simulink model "activity2_df1_uncorrected"  (R2024b)
settings: Solver=FixedStepAuto  StartTime=0.0  StopTime=10.0  FixedStep=1/44100  RelTol=1e-3
libraries: dspsnks4 x1, dspvision x1
settings Model: Creator=ck  LastModifiedBy=ck

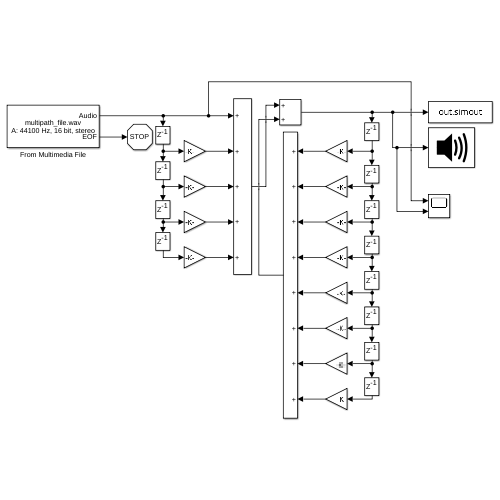
[thumbnail: Simulink's stored preview of the top-level diagram]
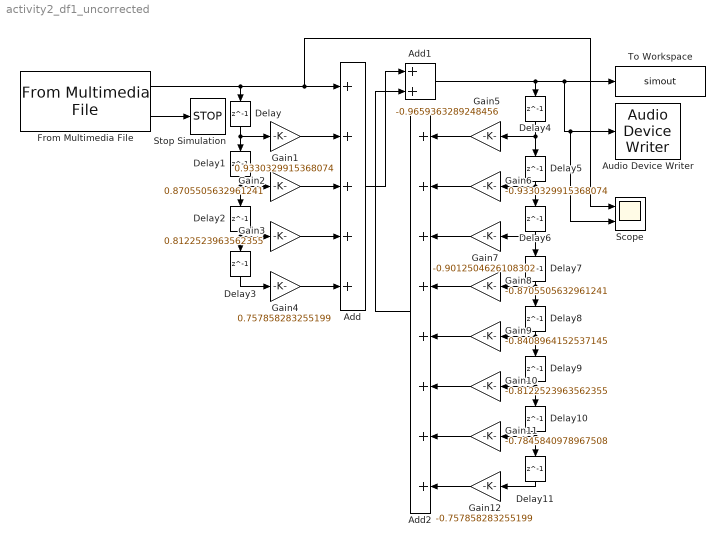
== system activity2_df1_uncorrected ==
  Add : Sum  Inputs=+++++
  Add1 : Sum
  Add2 : Sum  Inputs=++++++++
  Audio Device Writer : dspsnks4/Audio Device Writer  Driver=ALSA  Device=Default  InheritSampleRate=on  SampleRate=44100  BitDepth=16-bit integer  BufferSize=4096  NumBuffers=10  DefaultOutputChannelMapping=on  OutputChannelMapping=1:2  OutputNumUnderrunSamples=off  DriverIdx=8  DeviceWarnFlag=''
  Delay{,1..11} (12 alike) : Delay  DelayLength=1  InitialCondition=0
  From Multimedia File : dspvision/From Multimedia File  inputFilename=/home/ck/Documents/ece164/multipath_file.wav  readRange=[1 Inf]  loop=on  numPlays=inf  outputStreams=Audio only  videoDataType=single  audioDataType=double  inheritSampleTime=on  userDefinedSampleTime=1/30  noAudioOutput=off  isIntensityVideo=off  fourcc=RGB  colorVideoFormat=One multidimensional signal  outputEOF=on  dataOrg=Column-major  audioFrameSize=1  computeAudioFrameSize=off  outSamplingMode=Sample based
      settings: LibrarySourceBlock=dspsrcs4/From Multimedia File
  Gain1 : Gain  Gain=0.9330329915368074
  Gain10 : Gain  Gain=-0.8122523963562355
  Gain11 : Gain  Gain=-0.7845840978967508
  Gain12 : Gain  Gain=-0.757858283255199
  Gain2 : Gain  Gain=0.8705505632961241
  Gain3 : Gain  Gain=0.8122523963562355
  Gain4 : Gain  Gain=0.757858283255199
  Gain5 : Gain  Gain=-0.9659363289248456
  Gain6 : Gain  Gain=-0.9330329915368074
  Gain7 : Gain  Gain=-0.9012504626108302
  Gain8 : Gain  Gain=-0.8705505632961241
  Gain9 : Gain  Gain=-0.8408964152537145
  Scope : Scope  NumInputPorts=2
  Stop Simulation : Stop
  To Workspace : ToWorkspace  VariableName=simout  SaveFormat=Timeseries  SampleTime=-1
  wires:
  From Multimedia File/2 -> Stop Simulation/1
  From Multimedia File/1 -> Scope/1, Add/1, Delay/1
  Add/1 -> Add1/1
  Gain1/1 -> Add/2
  Gain2/1 -> Add/3
  Gain3/1 -> Add/4
  Gain4/1 -> Add/5
  Delay/1 -> Gain1/1, Delay1/1
  Delay1/1 -> Gain2/1, Delay2/1
  Delay2/1 -> Gain3/1, Delay3/1
  Delay3/1 -> Gain4/1
  Gain5/1 -> Add2/1
  Gain6/1 -> Add2/2
  Gain7/1 -> Add2/3
  Gain8/1 -> Add2/4
  Gain9/1 -> Add2/5
  Gain10/1 -> Add2/6
  Gain11/1 -> Add2/7
  Gain12/1 -> Add2/8
  Add2/1 -> Add1/2
  Delay5/1 -> Delay6/1, Gain6/1
  Delay6/1 -> Delay7/1, Gain7/1
  Delay9/1 -> Delay10/1, Gain10/1
  Delay10/1 -> Delay11/1, Gain11/1
  Delay8/1 -> Delay9/1, Gain9/1
  Delay7/1 -> Delay8/1, Gain8/1
  Delay11/1 -> Gain12/1
  Delay4/1 -> Delay5/1, Gain5/1
  Add1/1 -> Delay4/1, Scope/2, Audio Device Writer/1, To Workspace/1
